simulink model "ProyectoFinal_SC2"  (R2021a)
settings: Solver=VariableStepAuto  StartTime=0.0  StopTime=0.1  RelTol=1e-3
undefined symbols (not defined in the file): A, A_obs, Acl, B, B_obs, C, C_obs, D, D_obs, Klqr, Nbar, uss, xss
settings Model: Creator=fersa  LastModifiedBy=fersa

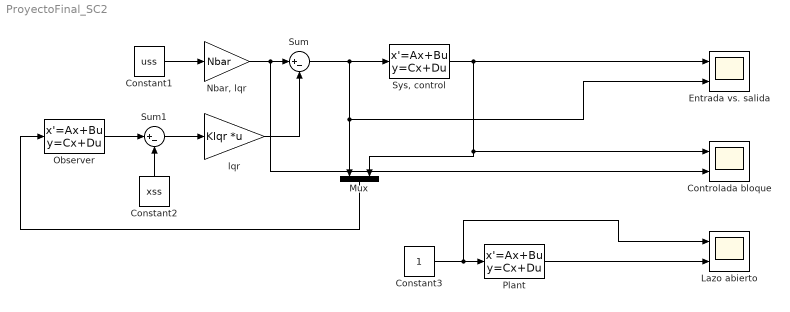
== system ProyectoFinal_SC2 ==
  Constant1 : Constant  Value=uss
  Constant2 : Constant  Value=xss
  Constant3 : Constant
  Controlada bloque : Scope  NumInputPorts=2
  Entrada vs. salida : Scope  NumInputPorts=2
  Lazo abierto : Scope  NumInputPorts=2
  Mux : Mux  Inputs=2
  "Nbar, lqr" : Gain  Gain=Nbar
  Observer : StateSpace  A=A_obs  B=B_obs  C=C_obs  D=D_obs  InitialCondition=0
  Plant : StateSpace  A=A  B=B  C=C  D=D  InitialCondition=0
  Sum : Sum  Inputs=|+-
  Sum1 : Sum  Inputs=|+-
  "Sys, control" : StateSpace  A=Acl  B=B  C=C  D=0  InitialCondition=0
  lqr : Gain  Gain=Klqr  Multiplication=Matrix(K*u) (u vector)
  wires:
  Constant1/1 -> "Nbar, lqr"/1
  "Nbar, lqr"/1 -> Controlada bloque/2, Sum/1
  lqr/1 -> Sum/2
  Sum1/1 -> lqr/1
  Constant2/1 -> Sum1/2
  Observer/1 -> Sum1/1
  Sum/1 -> "Sys, control"/1, Entrada vs. salida/2, Mux/1
  Constant3/1 -> Lazo abierto/1, Plant/1
  Mux/1 -> Observer/1
  "Sys, control"/1 -> Mux/2, Controlada bloque/1, Entrada vs. salida/1
  Plant/1 -> Lazo abierto/2
